simulink model "flanger"  (R2018a)
settings: Solver=FixedStepAuto  StartTime=0.0  StopTime=1.5  RelTol=1e-3  EnableMultiTasking=on
libraries: dspvision x2, dspsrcs4 x1
settings Model: Creator=Lu  LastModifiedBy=Lu
settings DebuggingCC: SingleTaskRateTransMsg=error

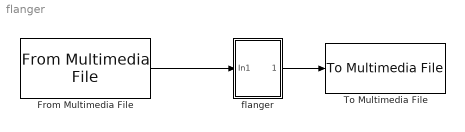
== system flanger ==
  From Multimedia File : dspvision/From Multimedia File  inputFilename=C:\Users\lugfe\Documents\GitHub\dsp-fpgay\TP FINAL\audio effects\test_flanger.wav  loop=on  numPlays=1  outputStreams=Audio only  videoDataType=single  audioDataType=int16  inheritSampleTime=on  userDefinedSampleTime=1/30  noAudioOutput=off  isIntensityVideo=off  fourcc=RGB  colorVideoFormat=Separate color signals  outputEOF=off  dataOrg=Column-major  audioFrameSize=1  computeAudioFrameSize=off  outSamplingMode=Sample based
      settings: SourceProductBaseCode=VP
  To Multimedia File : dspvision/To Multimedia File  outputFilename=C:\Users\lugfe\Documents\GitHub\dsp-fpgay\TP FINAL\audio effects\flanger_out.wav  streamSelection=Audio only  videoCompressor=None (uncompressed)  audioCompressor=None (uncompressed)  imagePorts=Separate color signals  fileType=WAV  audioDatatype=Determine from input data type  fourcc=RGB  videoQuality=75  mj2000CompFactor=10
      settings: SourceProductName=Computer Vision System Toolbox  SourceProductBaseCode=VP
  flanger : Subsystem
  wires:
  From Multimedia File/1 -> flanger/1(In1)
  flanger/1(Out1) -> To Multimedia File/1

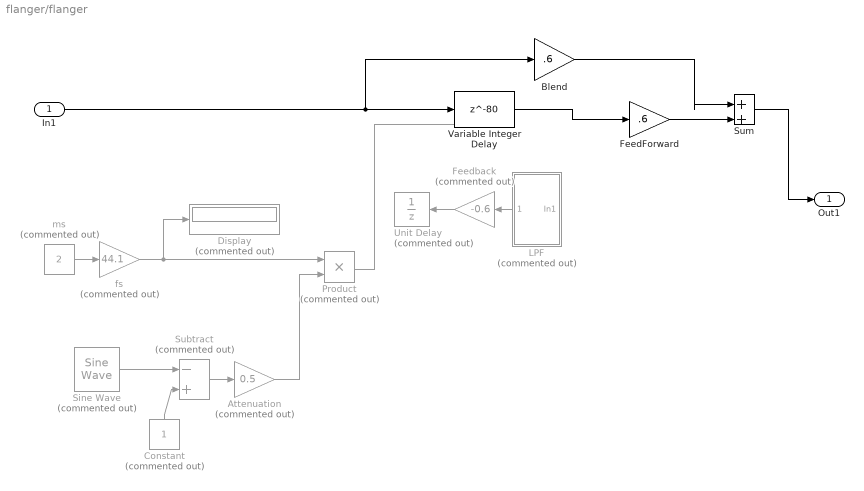
== system flanger/flanger ==
  In1 : Inport  OutDataTypeStr=int16  SampleTime=44100
  Attenuation : Gain  Commented=on  Gain=0.5  ParamDataTypeStr=int16  OutDataTypeStr=int16  RndMeth=Round
  Blend : Gain  Gain=.6  ParamDataTypeStr=int16  OutDataTypeStr=int16
  Constant : Constant  Commented=on  OutDataTypeStr=int16
  Display : Display  Commented=on
  FeedForward : Gain  Gain=.6  OutDataTypeStr=int16
  Feedback : Gain  Commented=on  Gain=-0.6  ParamDataTypeStr=int16  OutDataTypeStr=int16
  LPF : Subsystem  Commented=on
  Product : Product  Commented=on  OutDataTypeStr=int16  RndMeth=Round
  Sine Wave : dspsrcs4/Sine Wave  Commented=on  Amplitude=1  Frequency=1  Phase=0  SampleMode=Discrete  OutComplex=Real  CompMethod=Table lookup  TableSize=Speed  SampleTime=1/44100  SamplesPerFrame=1  ResetState=Restart at time zero  OutputFrames=off  dataType=Inherit via back propagation  wordLen=16  udDataType=sfix(16)  fracBitsMode=Best precision  numFracBits=15  OutDataTypeStr=Inherit: Inherit via back propagation  LastOutDataTypeStr=Inherit: Inherit via back propagation
  Subtract : Sum  Commented=on  Inputs=-+  AccumDataTypeStr=int16  OutDataTypeStr=int16  RndMeth=Round
  Sum : Sum  Inputs=|++  AccumDataTypeStr=int16
  Unit Delay : UnitDelay  Commented=on  InputProcessing=Columns as channels (frame based)  SampleTime=44100
  Variable Integer Delay : Delay  DelayLength=80  InputProcessing=Columns as channels (frame based)  SampleTime=44100
  fs : Gain  Commented=on  Gain=44.1
  ms : Constant  Commented=on  Value=2  OutDataTypeStr=int16
  Out1 : Outport  SampleTime=44100
  wires:
  Sum/1 -> Out1/1
  FeedForward/1 -> Sum/2
  Feedback/1 -> Unit Delay/1
  fs/1 -> Product/1, Display/1
  Constant/1 -> Subtract/2
  Sine Wave/1 -> Subtract/1
  Attenuation/1 -> Product/2
  Blend/1 -> Sum/1
  Subtract/1 -> Attenuation/1
  Variable Integer Delay/1 -> FeedForward/1
  LPF/1(Out1) -> Feedback/1
  In1/1 -> Variable Integer Delay/1, Blend/1
  ms/1 -> fs/1
  Product/1 -> ?

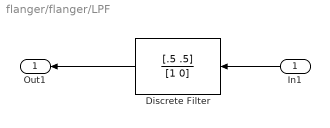
== system flanger/flanger/LPF ==
  In1 : Inport
  Discrete Filter : DiscreteFilter  Numerator=[.5 .5]  Denominator=[1 0]  InputProcessing=Columns as channels (frame based)  FilterStructure=Direct form II transposed  SampleTime=44100  a0EqualsOne=on  OutDataTypeStr=Inherit: Same as input
  Out1 : Outport
  wires:
  Discrete Filter/1 -> Out1/1
  In1/1 -> Discrete Filter/1
